simulink library "SUB_ECU_L4_MABX_HW_Interface"  (R2018a)
settings: Solver=VariableStepAuto  StartTime=0.0  StopTime=10.0  RelTol=1e-3
PostLoadFcn:
  | , if any(exist('dsrtsu_mdlpostloadfcn', 'file') == [2, 3, 6]), try dsrtsu_mdlpostloadfcn('Execute', bdroot); catch fprintf('Error in PostLoadFcn (dsrtsu_mdlpostloadfcn) for model "%s":\n %s\n', bdroot, lasterr); end, end,
undefined symbols (not defined in the file or in its folder): CANR_PROPB_REAX_3_13_CHANNEL_APV, CANR_PROPB_REAX_4_13_CHANNEL_APV, CANR_PROPB_XPR_1_50_CHANNEL_APV, ENUM_CAN_RX_T, ENUM_CAN_TX_T, ENUM_REAX_OPERATION_MODE_T, ENUM_SIGNAL_HEALTH_T, ENUM_XBR_CONTROL_MODE_T, ENUM_XBR_EBI_MODE_T, ENUM_XBR_PASS_THROUGH_ACTIVE_T, ENUM_XBR_PRIORITY_T, ENUM_XPR_INHIBIT_PARK_MANUAL_T, ENUM_XPR_INHIBIT_UNPARK_MANUAL_T, ENUM_XPR_PARK_MANUAL_T, ENUM_XPR_UNPARK_MANUAL_T, PROPB_REAX_1_E4_DES_POS_SIG_SRC_APV, PROPB_REAX_1_E4_DESIRED_OPMODE_APV, PROPB_REAX_1_E4_DESIRED_POSITION_APV, ptc_matlab_lib
libraries: PTC_MBDS_LIB x264, rtican x172, EmE_MBD_Blockset x39, simulink x34, $bdroot x16, rti1401lib_dio_type4 x8, simulink_need_slupdate x7, dsa_tcpip_lib x4, rti1401lib_adc_type4 x3, rtmapslib x3, rtitasklib x3
(part 29 of 51)

== system SUB_ECU_L4_MABX_HW_Interface/CAN_Truck1571/CAN_RX_PROPB_REAX_3_13/RX_CAN_1 ==
  Enable : Inport
  Bus Creator3 : BusCreator  Inputs=4
  CAN_TYPE1_RX_M1_C1 : rtican/RTICAN Receive (RX)   Reserved1=[]  Reserved2=[]  Reserved3=[]  Reserved4=[]  SfcnMessage=[]  Msg_Struct=[]  BoardTypeNo=[]  BoardNo=[]  ChannelNo=[]  Parameters=[]  DialogFcn=[]  UnitName=[]  Revision=[]  UnitValues=[]  DSProperties=struct('RTI',struct('Version',uint32(5),'BlockType',struct('isSLSource',uint8(1),'isSLSink',uint8(1),'isHWSource',uint8(0),'isHWSink',uint8(0),'isSetup',uint8(0),'isInline',uint8(1),'isNonInline',uint8(0),'isInterrupt',uint8(0),'isChannelwise',uint8(0)),'IOBoardType','RTICAN','UnitType','MESSAGE','Identifier','RX','DialogType','MSVC','BlockSet','RTICAN','SlaveProcessor','CAN'))  RTIBlockInterface=struct('OutputPortsWidth',int32([1 1 1 1 1 1 1 1 1 1 1]),'OutputPortsActive',ones(1,11),'OutputPortsName',{{'byte1','byte2','byte3','byte4','byte5','byte6','byte7','byte8',['RX status'],['RX time'],['RX delta time']}},'OutputPortsDataType',{{'SS_DOUBLE','SS_DOUBLE','SS_DOUBLE','SS_DOUBLE','SS_DOUBLE','SS_DOUBLE','SS_DOUBLE','SS_DOUBLE','SS_DOUBLE','SS_DOUBLE','SS_DOUBLE'}},'OutputPortsLabel',{{'byte1','byte2','byte3','byte4','byte5','byte6','byte7','byte8','','',''}},'OutputPortsLabelMode','ON','InputPortsWidth',int32(0),'InputPortsActive',0,'DialogFcn','rtican_message_interface_gui','BlockDisplay',{{'','center'}},'IconTransparency','on','ParameterTunableNames',{{}},'InitLevel',3,'BlockName',struct('Token',{{'CAN_TYPE','_RX_M','_C'}},'BlockParam',{{'BoardTypeNo','BoardNo','ChannelNo'}}),'SampleTime',{{-1}},'TriggerPort',{{'none'}},'EnablePort',{{'yes'}})  RTIBlockParameters=struct('BoardTypeNo',{{1,'OFF',[]}},'BoardNo',{{1,'ON',[1 16]}},'ChannelNo',{{1,'ON',[1 2]}},'Parameters',{{struct('DataFileSupport',struct('DataFileSelectedMaster',1,'DataFileSelectedLocal',0,'DataFileName',['c:\localdata\chris\advanced_tech\adas\ptc_autonomous_truck_secure\branches\truck1571\dbc\mabx_can1.dbc|c:\localdata\chris\advanced_tech\adas\ptc_autonomous_truck_secure\branches\svn\powertrainsys\trunk\src\projects_rcp\my2017_rcp\dbc files\j1939.dbc|'],'DataFileDate',{{{['04-Nov-2016 10:11:27']}}},'SelectedFile',['<no file selected>']),'Options',struct('StatusSelected',1,'TimeSelected',1,'DeltaTimeSelected',1,'BytePortSelected',0,'MessageLengthSelected',0,'TriggerPort',struct('Selected',0,'TriggerType',0),'UserCoding',struct('Selected',0,'InterfaceFile','UserDecodingFile','FcnName','UserDecodeFcn','InportSelected',0,'InportWidth',1,'OutportSelected',0,'OutportWidth',1),'EnablePortSelected',1,'SignalOnPortnameSelected',1,'UseRXService',1),'Message',struct('MsgOnBlocknameSelected',0,'MsgName','PropB_REAX_3_13','MsgIdFormat',1,'MsgId',419426579,'MsgLength',8,'NumSignals',8,'SampleTime',-1,'Signal',struct('SgnName',{'byte1','byte2','byte3','byte4','byte5','byte6','byte7','byte8'},'SgnStartBit',{0,8,16,24,32,40,48,56},'SgnLength',{8,8,8,8,8,8,8,8},'SgnType',{0,0,0,0,0,0,0,0},'ModeValue',{-1,-1,-1,-1,-1,-1,-1,-1},'DataType',{0,0,0,0,0,0,0,0},'ByteLayout',{0,0,0,0,0,0,0,0},'Factor',{1,1,1,1,1,1,1,1},'Offset',{0,0,0,0,0,0,0,0},'SgnComment',{{''},{''},{''},{''},{''},{''},{''},{''}},'SgnUnit',{'','','','','','','',''},'Min',{0,0,0,0,0,0,0,0},'Max',{0,0,0,0,0,0,0,0},'SLDataType',{'SS_DOUBLE','SS_DOUBLE','SS_DOUBLE','SS_DOUBLE','SS_DOUBLE','SS_DOUBLE','SS_DOUBLE','SS_DOUBLE'}),'MsgIdNumFormat',1,'MsgComment',{{['Response message B from TRW steering wheel']}}),'Version',1.2,'general',struct('isFromLib',0)),'OFF',[]}},'GroupId',{{struct('Group',{{'RTICAN'}},'No',7,'Behavior',{{'NAMECHANGE'}},'BlockType',{{'SINK'}},'NameChangeFlag',0),'OFF',[]}},'SFcnRTICANMessage',{{struct('MsgType','RX','SFcnPortType','Scalar','MsgName','PropB_REAX_3_13','MsgIdFormat','XTD','MsgId',419426579,'MsgLength',8,'NumSignals',8,'SampleTime',-1,'Signal',struct('SgnName',{'byte1','byte2','byte3','byte4','byte5','byte6','byte7','byte8'},'SgnStartBit',{0,8,16,24,32,40,48,56},'SgnLength',{8,8,8,8,8,8,8,8},'SgnType',{'standard','standard','standard','standard','standard','standard','standard','standard'},'ModeValue',{-1,-1,-1,-1,-1,-1,-1,-1},'DataType',{['unsigned int'],['unsigned int'],['unsigned int'],['unsigned int'],['unsigned int'],['unsigned int'],['unsigned int'],['unsigned int']},'ByteLayout',{['little endian'],['little endian'],['little endian'],['little endian'],['little endian'],['little endian'],['little endian'],['little endian']},'Factor',{1,1,1,1,1,1,1,1},'Offset',{0,0,0,0,0,0,0,0},'SLDataType',{'SS_DOUBLE','SS_DOUBLE','SS_DOUBLE','SS_DOUBLE','SS_DOUBLE','SS_DOUBLE','SS_DOUBLE','SS_DOUBLE'}),'StatusSelected','yes','TimeSelected','yes','DeltaTimeSelected','yes','BytePortSelected','no','MessageLengthSelected','no','TriggerPort',struct('Selected','no','TriggerType',0),'UserCoding',struct('Selected','no','InterfaceFile','UserDecodingFile','FcnName','UserDecodeFcn','InportSelected','no','InportWidth',1,'OutportSelected','no','OutportWidth',1),'EnablePortSelected','yes','UseRXService','yes','BoardType','DS1','BoardNo',1,'ControllerNo',1),'OFF',[]}},'TLCFileName',{{'rtican_rx_message','OFF',[]}})  RTISFcnParameters=struct('SFcnRTICANMessage','struct','TLCFileName','char')  RTIBlockParaDefault=struct('BoardTypeNo',4302,'BoardNo',1,'ChannelNo',1,'Parameters',struct('DataFileSupport',struct('DataFileSelectedMaster',0,'DataFileSelectedLocal',0,'DataFileName','','DataFileDate','','SelectedFile',['<no file selected>']),'Options',struct('StatusSelected',1,'TimeSelected',1,'DeltaTimeSelected',1,'BytePortSelected',0,'MessageLengthSelected',0,'TriggerPort',struct('Selected',0,'TriggerType','rising'),'UserCoding',struct('Selected',0,'InterfaceFile','UserDecodingFile','FcnName','UserDecodeFcn','InportSelected',0,'InportWidth',1,'OutportSelected',0,'OutportWidth',1),'EnablePortSelected',0,'SignalOnPortnameSelected',1,'UseRXService',0),'Message',struct('MsgOnBlocknameSelected',0,'MsgName',['RX Message'],'MsgIdFormat',0,'MsgId',100,'MsgLength',8,'NumSignals',1,'SampleTime',-1,'Signal',struct('SgnName',['RX signal'],'SgnStartBit',0,'SgnLength',8,'SgnType',0,'ModeValue',-1,'DataType',0,'SLDataType','SS_DOUBLE','ByteLayout',0,'Factor',1,'Offset',0,'Min',0,'Max',255,'SgnComment',{{}},'SgnUnit',''),'MsgIdNumFormat',0,'MsgComment',{{''}}),'Version',1.2,'general',struct('isFromLib',1)),'GroupId',struct('Group',{{'RTICAN'}},'No',1,'Behavior',{{'NAMECHANGE'}},'BlockType',{{'SINK'}},'NameChangeFlag',0),'SFcnRTICANMessage',struct('MsgType','RX','MsgName',['RX Message'],'MsgIdFormat','STD','MsgId',100,'MsgLength',8,'NumSignals',1,'SampleTime',-1,'Signal',struct('SgnName',['RX signal'],'SgnStartBit',0,'SgnLength',8,'SgnType','standard','ModeValue',-1,'DataType',['unsigned int'],'ByteLayout',['little endian'],'SLDataType','SS_DOUBLE','Factor',1,'Offset',0),'StatusSelected','yes','TimeSelected','yes','DeltaTimeSelected','yes','BytePortSelected','no','MessageLengthSelected','no','EnablePortSelected','no','UserCoding',struct('Selected','no','InterfaceFile','UserDecodingFile','FcnName','UserDecodeFcn','InportSelected','no','InportWidth',1,'OutportSelected','no','OutportWidth',1),'TriggerPort',struct('Selected','no','TriggerType','rising'),'UseRXService','no','BoardType','DS4302','BoardNo',1,'ControllerNo',1,'SFcnPortType','Scalar'),'TLCFileName','rtican_rx_message')
      settings: AttributesFormatString=Group Id: RTICAN7\n  SourceProductName=dSPACE RTI CAN Blockset
  Data Type Conversion{,1..7} (8 alike) : DataTypeConversion  OutDataTypeStr=uint8  SaturateOnIntegerOverflow=on
  Data Type Conversion10 : DataTypeConversion  OutDataTypeStr=double  SaturateOnIntegerOverflow=on
  Data Type Conversion8 : DataTypeConversion  OutDataTypeStr=boolean  SaturateOnIntegerOverflow=on
  Data Type Conversion9 : DataTypeConversion  OutDataTypeStr=double  SaturateOnIntegerOverflow=on
  Mux : Mux  Inputs=8
  PROPB_REAX_3_13 : Outport
  wires:
  Bus Creator3/1 -> PROPB_REAX_3_13/1  "PROPB_REAX_3_13"
  CAN_TYPE1_RX_M1_C1/1 -> Data Type Conversion/1  "byte1"
  CAN_TYPE1_RX_M1_C1/3 -> Data Type Conversion2/1  "byte3"
  CAN_TYPE1_RX_M1_C1/4 -> Data Type Conversion3/1  "byte4"
  CAN_TYPE1_RX_M1_C1/2 -> Data Type Conversion1/1  "byte2"
  CAN_TYPE1_RX_M1_C1/6 -> Data Type Conversion5/1  "byte6"
  CAN_TYPE1_RX_M1_C1/5 -> Data Type Conversion4/1  "byte5"
  CAN_TYPE1_RX_M1_C1/8 -> Data Type Conversion7/1  "byte8"
  CAN_TYPE1_RX_M1_C1/7 -> Data Type Conversion6/1  "byte7"
  Data Type Conversion3/1 -> Mux/4
  Data Type Conversion4/1 -> Mux/5
  Data Type Conversion2/1 -> Mux/3
  Data Type Conversion5/1 -> Mux/6
  Data Type Conversion1/1 -> Mux/2
  Data Type Conversion6/1 -> Mux/7
  Data Type Conversion/1 -> Mux/1
  Data Type Conversion7/1 -> Mux/8
  Mux/1 -> Bus Creator3/1  "RawData"
  Enable/1 -> CAN_TYPE1_RX_M1_C1/Enable
  CAN_TYPE1_RX_M1_C1/11 -> Data Type Conversion10/1
  CAN_TYPE1_RX_M1_C1/10 -> Data Type Conversion9/1
  CAN_TYPE1_RX_M1_C1/9 -> Data Type Conversion8/1
  Data Type Conversion8/1 -> Bus Creator3/2  "RX_status"
  Data Type Conversion10/1 -> Bus Creator3/4  "RX_delta_time"
  Data Type Conversion9/1 -> Bus Creator3/3  "RX_time"

== system SUB_ECU_L4_MABX_HW_Interface/CAN_Truck1571/CAN_RX_PROPB_REAX_3_13/SelectChannel ==
  In1 : Inport
  Constant : Constant  Value=ENUM_CAN_RX_T.RX_CAN_1
  Constant1 : Constant  Value=ENUM_CAN_RX_T.RX_CAN_2
  Constant2 : Constant  Value=ENUM_CAN_RX_T.RX_CAN_3
  Constant3 : Constant  Value=ENUM_CAN_RX_T.RX_CAN_4
  Constant4 : Constant  Value=ENUM_CAN_RX_T.RX_CAN_5
  Constant5 : Constant  Value=ENUM_CAN_RX_T.RX_CAN_6
  EQ{,1..5} (6 alike) : PTC_MBDS_LIB/MBDS Standard Library/Basic Operations/Logic and Bit Operations/EQ  InputSameDT=on  PTC_MBDS_BlockVersion=5.41  PTC_BlockType=PTC_MBDS_EQ
      settings: SourceProductName=PACCAR Technical Center MBDS Library
  CAN1 : Outport
  CAN2 : Outport  Port=2
  CAN3 : Outport  Port=3
  CAN4 : Outport  Port=4
  CAN5 : Outport  Port=5
  CAN6 : Outport  Port=6
  wires:
  In1/1 -> EQ5/1, EQ4/1, EQ3/1, EQ2/1, EQ1/1, EQ/1
  Constant/1 -> EQ/2
  EQ/1 -> CAN1/1
  Constant1/1 -> EQ1/2
  Constant2/1 -> EQ2/2
  Constant3/1 -> EQ3/2
  Constant4/1 -> EQ4/2
  Constant5/1 -> EQ5/2
  EQ1/1 -> CAN2/1
  EQ2/1 -> CAN3/1
  EQ3/1 -> CAN4/1
  EQ4/1 -> CAN5/1
  EQ5/1 -> CAN6/1

== system SUB_ECU_L4_MABX_HW_Interface/CAN_Truck1571/CAN_RX_PROPB_REAX_4_13/RX_CAN_1 ==
  Enable : Inport
  Bus Creator3 : BusCreator  Inputs=4
  CAN_TYPE1_RX_M1_C1 : rtican/RTICAN Receive (RX)   Reserved1=[]  Reserved2=[]  Reserved3=[]  Reserved4=[]  SfcnMessage=[]  Msg_Struct=[]  BoardTypeNo=[]  BoardNo=[]  ChannelNo=[]  Parameters=[]  DialogFcn=[]  UnitName=[]  Revision=[]  UnitValues=[]  DSProperties=struct('RTI',struct('Version',uint32(5),'BlockType',struct('isSLSource',uint8(1),'isSLSink',uint8(1),'isHWSource',uint8(0),'isHWSink',uint8(0),'isSetup',uint8(0),'isInline',uint8(1),'isNonInline',uint8(0),'isInterrupt',uint8(0),'isChannelwise',uint8(0)),'IOBoardType','RTICAN','UnitType','MESSAGE','Identifier','RX','DialogType','MSVC','BlockSet','RTICAN','SlaveProcessor','CAN'))  RTIBlockInterface=struct('OutputPortsWidth',int32([1 1 1 1 1 1 1 1 1 1 1]),'OutputPortsActive',ones(1,11),'OutputPortsName',{{'byte1','byte2','byte3','byte4','byte5','byte6','byte7','byte8',['RX status'],['RX time'],['RX delta time']}},'OutputPortsDataType',{{'SS_DOUBLE','SS_DOUBLE','SS_DOUBLE','SS_DOUBLE','SS_DOUBLE','SS_DOUBLE','SS_DOUBLE','SS_DOUBLE','SS_DOUBLE','SS_DOUBLE','SS_DOUBLE'}},'OutputPortsLabel',{{'byte1','byte2','byte3','byte4','byte5','byte6','byte7','byte8','','',''}},'OutputPortsLabelMode','ON','InputPortsWidth',int32(0),'InputPortsActive',0,'DialogFcn','rtican_message_interface_gui','BlockDisplay',{{'','center'}},'IconTransparency','on','ParameterTunableNames',{{}},'InitLevel',3,'BlockName',struct('Token',{{'CAN_TYPE','_RX_M','_C'}},'BlockParam',{{'BoardTypeNo','BoardNo','ChannelNo'}}),'SampleTime',{{-1}},'TriggerPort',{{'none'}},'EnablePort',{{'yes'}})  RTIBlockParameters=struct('BoardTypeNo',{{1,'OFF',[]}},'BoardNo',{{1,'ON',[1 16]}},'ChannelNo',{{1,'ON',[1 2]}},'Parameters',{{struct('DataFileSupport',struct('DataFileSelectedMaster',1,'DataFileSelectedLocal',0,'DataFileName','c:\data\svn\ptc_autonomous_truck_secure\trunk\candb\selfdrivingtruck.dbc|','DataFileDate',{{{['04-Nov-2016 10:11:27']}}},'SelectedFile',['<no file selected>']),'Options',struct('StatusSelected',1,'TimeSelected',1,'DeltaTimeSelected',1,'BytePortSelected',0,'MessageLengthSelected',0,'TriggerPort',struct('Selected',0,'TriggerType',0),'UserCoding',struct('Selected',0,'InterfaceFile','UserDecodingFile','FcnName','UserDecodeFcn','InportSelected',0,'InportWidth',1,'OutportSelected',0,'OutportWidth',1),'EnablePortSelected',1,'SignalOnPortnameSelected',1,'UseRXService',1),'Message',struct('MsgOnBlocknameSelected',0,'MsgName','PropB_REAX_4_13','MsgIdFormat',1,'MsgId',419428115,'MsgLength',8,'NumSignals',8,'SampleTime',-1,'Signal',struct('SgnName',{'byte1','byte2','byte3','byte4','byte5','byte6','byte7','byte8'},'SgnStartBit',{0,8,16,24,32,40,48,56},'SgnLength',{8,8,8,8,8,8,8,8},'SgnType',{0,0,0,0,0,0,0,0},'ModeValue',{-1,-1,-1,-1,-1,-1,-1,-1},'DataType',{0,0,0,0,0,0,0,0},'ByteLayout',{0,0,0,0,0,0,0,0},'Factor',{1,1,1,1,1,1,1,1},'Offset',{0,0,0,0,0,0,0,0},'SgnComment',{{''},{''},{''},{''},{''},{''},{''},{''}},'SgnUnit',{'','','','','','','',''},'Min',{0,0,0,0,0,0,0,0},'Max',{0,0,0,0,0,0,0,0},'SLDataType',{'SS_DOUBLE','SS_DOUBLE','SS_DOUBLE','SS_DOUBLE','SS_DOUBLE','SS_DOUBLE','SS_DOUBLE','SS_DOUBLE'}),'MsgIdNumFormat',1,'MsgComment',{{['TRW diagnostic message']}}),'Version',1.2,'general',struct('isFromLib',0)),'OFF',[]}},'GroupId',{{struct('Group',{{'RTICAN'}},'No',7,'Behavior',{{'NAMECHANGE'}},'BlockType',{{'SINK'}},'NameChangeFlag',0),'OFF',[]}},'SFcnRTICANMessage',{{struct('MsgType','RX','SFcnPortType','Scalar','MsgName','PropB_REAX_4_13','MsgIdFormat','XTD','MsgId',419428115,'MsgLength',8,'NumSignals',8,'SampleTime',-1,'Signal',struct('SgnName',{'byte1','byte2','byte3','byte4','byte5','byte6','byte7','byte8'},'SgnStartBit',{0,8,16,24,32,40,48,56},'SgnLength',{8,8,8,8,8,8,8,8},'SgnType',{'standard','standard','standard','standard','standard','standard','standard','standard'},'ModeValue',{-1,-1,-1,-1,-1,-1,-1,-1},'DataType',{['unsigned int'],['unsigned int'],['unsigned int'],['unsigned int'],['unsigned int'],['unsigned int'],['unsigned int'],['unsigned int']},'ByteLayout',{['little endian'],['little endian'],['little endian'],['little endian'],['little endian'],['little endian'],['little endian'],['little endian']},'Factor',{1,1,1,1,1,1,1,1},'Offset',{0,0,0,0,0,0,0,0},'SLDataType',{'SS_DOUBLE','SS_DOUBLE','SS_DOUBLE','SS_DOUBLE','SS_DOUBLE','SS_DOUBLE','SS_DOUBLE','SS_DOUBLE'}),'StatusSelected','yes','TimeSelected','yes','DeltaTimeSelected','yes','BytePortSelected','no','MessageLengthSelected','no','TriggerPort',struct('Selected','no','TriggerType',0),'UserCoding',struct('Selected','no','InterfaceFile','UserDecodingFile','FcnName','UserDecodeFcn','InportSelected','no','InportWidth',1,'OutportSelected','no','OutportWidth',1),'EnablePortSelected','yes','UseRXService','yes','BoardType','DS1','BoardNo',1,'ControllerNo',1),'OFF',[]}},'TLCFileName',{{'rtican_rx_message','OFF',[]}})  RTISFcnParameters=struct('SFcnRTICANMessage','struct','TLCFileName','char')  RTIBlockParaDefault=struct('BoardTypeNo',4302,'BoardNo',1,'ChannelNo',1,'Parameters',struct('DataFileSupport',struct('DataFileSelectedMaster',0,'DataFileSelectedLocal',0,'DataFileName','','DataFileDate','','SelectedFile',['<no file selected>']),'Options',struct('StatusSelected',1,'TimeSelected',1,'DeltaTimeSelected',1,'BytePortSelected',0,'MessageLengthSelected',0,'TriggerPort',struct('Selected',0,'TriggerType','rising'),'UserCoding',struct('Selected',0,'InterfaceFile','UserDecodingFile','FcnName','UserDecodeFcn','InportSelected',0,'InportWidth',1,'OutportSelected',0,'OutportWidth',1),'EnablePortSelected',0,'SignalOnPortnameSelected',1,'UseRXService',0),'Message',struct('MsgOnBlocknameSelected',0,'MsgName',['RX Message'],'MsgIdFormat',0,'MsgId',100,'MsgLength',8,'NumSignals',1,'SampleTime',-1,'Signal',struct('SgnName',['RX signal'],'SgnStartBit',0,'SgnLength',8,'SgnType',0,'ModeValue',-1,'DataType',0,'SLDataType','SS_DOUBLE','ByteLayout',0,'Factor',1,'Offset',0,'Min',0,'Max',255,'SgnComment',{{}},'SgnUnit',''),'MsgIdNumFormat',0,'MsgComment',{{''}}),'Version',1.2,'general',struct('isFromLib',1)),'GroupId',struct('Group',{{'RTICAN'}},'No',1,'Behavior',{{'NAMECHANGE'}},'BlockType',{{'SINK'}},'NameChangeFlag',0),'SFcnRTICANMessage',struct('MsgType','RX','MsgName',['RX Message'],'MsgIdFormat','STD','MsgId',100,'MsgLength',8,'NumSignals',1,'SampleTime',-1,'Signal',struct('SgnName',['RX signal'],'SgnStartBit',0,'SgnLength',8,'SgnType','standard','ModeValue',-1,'DataType',['unsigned int'],'ByteLayout',['little endian'],'SLDataType','SS_DOUBLE','Factor',1,'Offset',0),'StatusSelected','yes','TimeSelected','yes','DeltaTimeSelected','yes','BytePortSelected','no','MessageLengthSelected','no','EnablePortSelected','no','UserCoding',struct('Selected','no','InterfaceFile','UserDecodingFile','FcnName','UserDecodeFcn','InportSelected','no','InportWidth',1,'OutportSelected','no','OutportWidth',1),'TriggerPort',struct('Selected','no','TriggerType','rising'),'UseRXService','no','BoardType','DS4302','BoardNo',1,'ControllerNo',1,'SFcnPortType','Scalar'),'TLCFileName','rtican_rx_message')
      settings: AttributesFormatString=Group Id: RTICAN7\n  SourceProductName=dSPACE RTI CAN Blockset
  Data Type Conversion{,1..7} (8 alike) : DataTypeConversion  OutDataTypeStr=uint8  SaturateOnIntegerOverflow=on
  Data Type Conversion10 : DataTypeConversion  OutDataTypeStr=double  SaturateOnIntegerOverflow=on
  Data Type Conversion8 : DataTypeConversion  OutDataTypeStr=boolean  SaturateOnIntegerOverflow=on
  Data Type Conversion9 : DataTypeConversion  OutDataTypeStr=double  SaturateOnIntegerOverflow=on
  Mux : Mux  Inputs=8
  PROPB_REAX_4_13 : Outport
  wires:
  Data Type Conversion9/1 -> Bus Creator3/3  "RX_time"
  Data Type Conversion10/1 -> Bus Creator3/4  "RX_delta_time"
  Data Type Conversion8/1 -> Bus Creator3/2  "RX_status"
  CAN_TYPE1_RX_M1_C1/9 -> Data Type Conversion8/1
  CAN_TYPE1_RX_M1_C1/10 -> Data Type Conversion9/1
  CAN_TYPE1_RX_M1_C1/11 -> Data Type Conversion10/1
  Enable/1 -> CAN_TYPE1_RX_M1_C1/Enable
  Mux/1 -> Bus Creator3/1  "RawData"
  Data Type Conversion7/1 -> Mux/8
  Data Type Conversion/1 -> Mux/1
  Data Type Conversion6/1 -> Mux/7
  Data Type Conversion1/1 -> Mux/2
  Data Type Conversion5/1 -> Mux/6
  Data Type Conversion2/1 -> Mux/3
  Data Type Conversion4/1 -> Mux/5
  Data Type Conversion3/1 -> Mux/4
  CAN_TYPE1_RX_M1_C1/7 -> Data Type Conversion6/1  "byte7"
  CAN_TYPE1_RX_M1_C1/8 -> Data Type Conversion7/1  "byte8"
  CAN_TYPE1_RX_M1_C1/5 -> Data Type Conversion4/1  "byte5"
  CAN_TYPE1_RX_M1_C1/6 -> Data Type Conversion5/1  "byte6"
  CAN_TYPE1_RX_M1_C1/2 -> Data Type Conversion1/1  "byte2"
  CAN_TYPE1_RX_M1_C1/4 -> Data Type Conversion3/1  "byte4"
  CAN_TYPE1_RX_M1_C1/3 -> Data Type Conversion2/1  "byte3"
  CAN_TYPE1_RX_M1_C1/1 -> Data Type Conversion/1  "byte1"
  Bus Creator3/1 -> PROPB_REAX_4_13/1  "PROPB_REAX_4_13"

== system SUB_ECU_L4_MABX_HW_Interface/CAN_Truck1571/CAN_RX_PROPB_REAX_4_13/SelectChannel ==
  In1 : Inport
  Constant : Constant  Value=ENUM_CAN_RX_T.RX_CAN_1
  Constant1 : Constant  Value=ENUM_CAN_RX_T.RX_CAN_2
  Constant2 : Constant  Value=ENUM_CAN_RX_T.RX_CAN_3
  Constant3 : Constant  Value=ENUM_CAN_RX_T.RX_CAN_4
  Constant4 : Constant  Value=ENUM_CAN_RX_T.RX_CAN_5
  Constant5 : Constant  Value=ENUM_CAN_RX_T.RX_CAN_6
  EQ{,1..5} (6 alike) : PTC_MBDS_LIB/MBDS Standard Library/Basic Operations/Logic and Bit Operations/EQ  InputSameDT=on  PTC_MBDS_BlockVersion=5.41  PTC_BlockType=PTC_MBDS_EQ
      settings: SourceProductName=PACCAR Technical Center MBDS Library
  CAN1 : Outport
  CAN2 : Outport  Port=2
  CAN3 : Outport  Port=3
  CAN4 : Outport  Port=4
  CAN5 : Outport  Port=5
  CAN6 : Outport  Port=6
  wires:
  EQ5/1 -> CAN6/1
  EQ4/1 -> CAN5/1
  EQ3/1 -> CAN4/1
  EQ2/1 -> CAN3/1
  EQ1/1 -> CAN2/1
  Constant5/1 -> EQ5/2
  Constant4/1 -> EQ4/2
  Constant3/1 -> EQ3/2
  Constant2/1 -> EQ2/2
  Constant1/1 -> EQ1/2
  EQ/1 -> CAN1/1
  Constant/1 -> EQ/2
  In1/1 -> EQ/1, EQ1/1, EQ2/1, EQ3/1, EQ4/1, EQ5/1

== system SUB_ECU_L4_MABX_HW_Interface/CAN_Truck1571/CAN_RX_PROPB_XPR_1_50/RX_CAN_1 ==
  Enable : Inport
  Bus Creator3 : BusCreator  Inputs=5
  CAN_TYPE1_RX_M1_C1 : rtican/RTICAN Receive (RX)   Reserved1=[]  Reserved2=[]  Reserved3=[]  Reserved4=[]  SfcnMessage=[]  Msg_Struct=[]  BoardTypeNo=[]  BoardNo=[]  ChannelNo=[]  Parameters=[]  DialogFcn=[]  UnitName=[]  Revision=[]  UnitValues=[]  DSProperties=struct('RTI',struct('Version',uint32(5),'BlockType',struct('isSLSource',uint8(1),'isSLSink',uint8(1),'isHWSource',uint8(0),'isHWSink',uint8(0),'isSetup',uint8(0),'isInline',uint8(1),'isNonInline',uint8(0),'isInterrupt',uint8(0),'isChannelwise',uint8(0)),'IOBoardType','RTICAN','UnitType','MESSAGE','Identifier','RX','DialogType','MSVC','BlockSet','RTICAN','SlaveProcessor','CAN'))  RTIBlockInterface=struct('OutputPortsWidth',int32([1 1 1 1 1]),'OutputPortsActive',[1 1 1 1 1],'OutputPortsName',{{'EPBPCMInhibitStatusFeedback','EPBPCMManualStatusFeedback',['RX status'],['RX time'],['RX delta time']}},'OutputPortsDataType',{{'SS_DOUBLE','SS_DOUBLE','SS_DOUBLE','SS_DOUBLE','SS_DOUBLE'}},'OutputPortsLabel',{{'EPBPCMInhibitStatusFeedback','EPBPCMManualStatusFeedback','','',''}},'OutputPortsLabelMode','ON','InputPortsWidth',int32(0),'InputPortsActive',0,'DialogFcn','rtican_message_interface_gui','BlockDisplay',{{'','center'}},'IconTransparency','on','ParameterTunableNames',{{}},'InitLevel',3,'BlockName',struct('Token',{{'CAN_TYPE','_RX_M','_C'}},'BlockParam',{{'BoardTypeNo','BoardNo','ChannelNo'}}),'SampleTime',{{-1}},'TriggerPort',{{'none'}},'EnablePort',{{'yes'}})  RTIBlockParameters=struct('BoardTypeNo',{{1,'OFF',[]}},'BoardNo',{{1,'ON',[1 16]}},'ChannelNo',{{1,'ON',[1 2]}},'Parameters',{{struct('DataFileSupport',struct('DataFileSelectedMaster',1,'DataFileSelectedLocal',0,'DataFileName',['c:\data\truck1571\dbc\mabx_can1.dbc|c:\data\svn\powertrainsys\trunk\src\projects_rcp\my2017_rcp\dbc files\j1939.dbc|'],'DataFileDate',{{{['04-Nov-2016 10:11:27']}}},'SelectedFile',['<no file selected>']),'Options',struct('StatusSelected',1,'TimeSelected',1,'DeltaTimeSelected',1,'BytePortSelected',0,'MessageLengthSelected',0,'TriggerPort',struct('Selected',0,'TriggerType',0),'UserCoding',struct('Selected',0,'InterfaceFile','UserDecodingFile','FcnName','UserDecodeFcn','InportSelected',0,'InportWidth',1,'OutportSelected',0,'OutportWidth',1),'EnablePortSelected',1,'SignalOnPortnameSelected',1,'UseRXService',1),'Message',struct('MsgOnBlocknameSelected',0,'MsgName','PropB_XPR_1','MsgIdFormat',1,'MsgId',419387472,'MsgLength',8,'NumSignals',2,'SampleTime',-1,'Signal',struct('SgnName',{'EPBPCMInhibitStatusFeedback','EPBPCMManualStatusFeedback'},'SgnStartBit',{0,2},'SgnLength',{2,2},'SgnType',{0,0},'ModeValue',{-1,-1},'DataType',{0,0},'ByteLayout',{0,0},'Factor',{1,1},'Offset',{0,0},'SgnComment',{{''},{''}},'SgnUnit',{'enum','enum'},'Min',{0,0},'Max',{0,0},'SLDataType',{'SS_DOUBLE','SS_DOUBLE'}),'MsgIdNumFormat',1,'MsgComment',{{['PropB XPR Feedback']}}),'Version',1.2,'general',struct('isFromLib',0)),'OFF',[]}},'GroupId',{{struct('Group',{{'RTICAN'}},'No',7,'Behavior',{{'NAMECHANGE'}},'BlockType',{{'SINK'}},'NameChangeFlag',0),'OFF',[]}},'SFcnRTICANMessage',{{struct('MsgType','RX','SFcnPortType','Scalar','MsgName','PropB_XPR_1','MsgIdFormat','XTD','MsgId',419387472,'MsgLength',8,'NumSignals',2,'SampleTime',-1,'Signal',struct('SgnName',{'EPBPCMInhibitStatusFeedback','EPBPCMManualStatusFeedback'},'SgnStartBit',{0,2},'SgnLength',{2,2},'SgnType',{'standard','standard'},'ModeValue',{-1,-1},'DataType',{['unsigned int'],['unsigned int']},'ByteLayout',{['little endian'],['little endian']},'Factor',{1,1},'Offset',{0,0},'SLDataType',{'SS_DOUBLE','SS_DOUBLE'}),'StatusSelected','yes','TimeSelected','yes','DeltaTimeSelected','yes','BytePortSelected','no','MessageLengthSelected','no','TriggerPort',struct('Selected','no','TriggerType',0),'UserCoding',struct('Selected','no','InterfaceFile','UserDecodingFile','FcnName','UserDecodeFcn','InportSelected','no','InportWidth',1,'OutportSelected','no','OutportWidth',1),'EnablePortSelected','yes','UseRXService','yes','BoardType','DS1','BoardNo',1,'ControllerNo',1),'OFF',[]}},'TLCFileName',{{'rtican_rx_message','OFF',[]}})  RTISFcnParameters=struct('SFcnRTICANMessage','struct','TLCFileName','char')  RTIBlockParaDefault=struct('BoardTypeNo',4302,'BoardNo',1,'ChannelNo',1,'Parameters',struct('DataFileSupport',struct('DataFileSelectedMaster',0,'DataFileSelectedLocal',0,'DataFileName','','DataFileDate','','SelectedFile',['<no file selected>']),'Options',struct('StatusSelected',1,'TimeSelected',1,'DeltaTimeSelected',1,'BytePortSelected',0,'MessageLengthSelected',0,'TriggerPort',struct('Selected',0,'TriggerType','rising'),'UserCoding',struct('Selected',0,'InterfaceFile','UserDecodingFile','FcnName','UserDecodeFcn','InportSelected',0,'InportWidth',1,'OutportSelected',0,'OutportWidth',1),'EnablePortSelected',0,'SignalOnPortnameSelected',1,'UseRXService',0),'Message',struct('MsgOnBlocknameSelected',0,'MsgName',['RX Message'],'MsgIdFormat',0,'MsgId',100,'MsgLength',8,'NumSignals',1,'SampleTime',-1,'Signal',struct('SgnName',['RX signal'],'SgnStartBit',0,'SgnLength',8,'SgnType',0,'ModeValue',-1,'DataType',0,'SLDataType','SS_DOUBLE','ByteLayout',0,'Factor',1,'Offset',0,'Min',0,'Max',255,'SgnComment',{{}},'SgnUnit',''),'MsgIdNumFormat',0,'MsgComment',{{''}}),'Version',1.2,'general',struct('isFromLib',1)),'GroupId',struct('Group',{{'RTICAN'}},'No',1,'Behavior',{{'NAMECHANGE'}},'BlockType',{{'SINK'}},'NameChangeFlag',0),'SFcnRTICANMessage',struct('MsgType','RX','MsgName',['RX Message'],'MsgIdFormat','STD','MsgId',100,'MsgLength',8,'NumSignals',1,'SampleTime',-1,'Signal',struct('SgnName',['RX signal'],'SgnStartBit',0,'SgnLength',8,'SgnType','standard','ModeValue',-1,'DataType',['unsigned int'],'ByteLayout',['little endian'],'SLDataType','SS_DOUBLE','Factor',1,'Offset',0),'StatusSelected','yes','TimeSelected','yes','DeltaTimeSelected','yes','BytePortSelected','no','MessageLengthSelected','no','EnablePortSelected','no','UserCoding',struct('Selected','no','InterfaceFile','UserDecodingFile','FcnName','UserDecodeFcn','InportSelected','no','InportWidth',1,'OutportSelected','no','OutportWidth',1),'TriggerPort',struct('Selected','no','TriggerType','rising'),'UseRXService','no','BoardType','DS4302','BoardNo',1,'ControllerNo',1,'SFcnPortType','Scalar'),'TLCFileName','rtican_rx_message')
      settings: AttributesFormatString=Group Id: RTICAN7\n  SourceProductName=dSPACE RTI CAN Blockset
  Data Type Conversion : DataTypeConversion  OutDataTypeStr=uint8  SaturateOnIntegerOverflow=on
  Data Type Conversion1 : DataTypeConversion  OutDataTypeStr=uint8  SaturateOnIntegerOverflow=on
  Data Type Conversion10 : DataTypeConversion  OutDataTypeStr=double  SaturateOnIntegerOverflow=on
  Data Type Conversion8 : DataTypeConversion  OutDataTypeStr=boolean  SaturateOnIntegerOverflow=on
  Data Type Conversion9 : DataTypeConversion  OutDataTypeStr=double  SaturateOnIntegerOverflow=on
  Data Type Conversion2 : DataTypeConversion  OutDataTypeStr=Enum: ENUM_XPR_FEEDBACK_T
      settings: AttributesFormatString=%<OutDataTypeStr>
  Data Type Conversion3 : DataTypeConversion  OutDataTypeStr=Enum: ENUM_XPR_FEEDBACK_T
      settings: AttributesFormatString=%<OutDataTypeStr>
  PROPB_XPR_1_50 : Outport
  wires:
  Data Type Conversion3/1 -> Bus Creator3/2  "EPBPCMManualStatusFeedback"
  Data Type Conversion2/1 -> Bus Creator3/1  "EPBPCMInhibitStatusFeedback"
  Data Type Conversion1/1 -> Data Type Conversion3/1
  Data Type Conversion/1 -> Data Type Conversion2/1
  CAN_TYPE1_RX_M1_C1/1 -> Data Type Conversion/1
  CAN_TYPE1_RX_M1_C1/2 -> Data Type Conversion1/1
  Data Type Conversion9/1 -> Bus Creator3/4  "RX_time"
  Data Type Conversion10/1 -> Bus Creator3/5  "RX_delta_time"
  Data Type Conversion8/1 -> Bus Creator3/3  "RX_status"
  CAN_TYPE1_RX_M1_C1/3 -> Data Type Conversion8/1
  CAN_TYPE1_RX_M1_C1/4 -> Data Type Conversion9/1
  CAN_TYPE1_RX_M1_C1/5 -> Data Type Conversion10/1
  Enable/1 -> CAN_TYPE1_RX_M1_C1/Enable
  Bus Creator3/1 -> PROPB_XPR_1_50/1  "PROPB_XPR_1_50"

== system SUB_ECU_L4_MABX_HW_Interface/CAN_Truck1571/CAN_RX_PROPB_XPR_1_50/SelectChannel ==
  In1 : Inport
  Constant : Constant  Value=ENUM_CAN_RX_T.RX_CAN_1
  Constant1 : Constant  Value=ENUM_CAN_RX_T.RX_CAN_2
  Constant2 : Constant  Value=ENUM_CAN_RX_T.RX_CAN_3
  Constant3 : Constant  Value=ENUM_CAN_RX_T.RX_CAN_4
  Constant4 : Constant  Value=ENUM_CAN_RX_T.RX_CAN_5
  Constant5 : Constant  Value=ENUM_CAN_RX_T.RX_CAN_6
  EQ{,1..5} (6 alike) : PTC_MBDS_LIB/MBDS Standard Library/Basic Operations/Logic and Bit Operations/EQ  InputSameDT=on  PTC_MBDS_BlockVersion=5.41  PTC_BlockType=PTC_MBDS_EQ
      settings: SourceProductName=PACCAR Technical Center MBDS Library
  CAN1 : Outport
  CAN2 : Outport  Port=2
  CAN3 : Outport  Port=3
  CAN4 : Outport  Port=4
  CAN5 : Outport  Port=5
  CAN6 : Outport  Port=6
  wires:
  EQ5/1 -> CAN6/1
  EQ4/1 -> CAN5/1
  EQ3/1 -> CAN4/1
  EQ2/1 -> CAN3/1
  EQ1/1 -> CAN2/1
  Constant5/1 -> EQ5/2
  Constant4/1 -> EQ4/2
  Constant3/1 -> EQ3/2
  Constant2/1 -> EQ2/2
  Constant1/1 -> EQ1/2
  EQ/1 -> CAN1/1
  Constant/1 -> EQ/2
  In1/1 -> EQ/1, EQ1/1, EQ2/1, EQ3/1, EQ4/1, EQ5/1
